simulink model "sampleModel25"  (Simulink 9.1)
settings: Solver=VariableStepAuto  StartTime=0.0  StopTime=10.0  RelTol=1e-3
undefined symbols (not defined in the file): DiscIntNeverNeededParam, Newton, Raphson
libraries: simulink x56
(part 1 of 2)
settings Model: SuppressorTable="22 serialization::archive 11 0 6 0 0 2 8 0 0 0 0 6 0 0 1 0 21 sampleModel25/cfblk71 0 6 0 0 2 8 0 0 0 0 6 41 Simulink:DataType:WarningOverFlowDetected 0 0 0 6 0  0  0 0 0 0 8 20160523 0 0 0 10 57 55 0 1 40 SimulinkFixedPoint:util:Overflowoccurred 0 0 0  0  8 20160523 0 10 57 55 0 1 1 0 21 sampleModel25/cfblk75 2 8 0 41 Simulink:DataType:WarningOverFlowDetected 0 0 0  0  8 20160608 0 15 23 17 0 1 40 SimulinkFixedPoint:util:Overflowoccurred 0 0 0  0  8 20160608 0 15 23 17 0 1"  Creator=DELL  LastModifiedBy=DELL
settings DataIOCC: SaveFormat=Dataset
settings OptimizationCC: LifeSpan=auto
settings DebuggingCC: UnderspecifiedInitializationDetection=Simplified  MergeDetectMultiDrivingBlocksExec=error  SFUnexpectedBacktrackingDiag=error  SFNoUnconditionalDefaultTransitionDiag=error  SFExecutionAtInitializationDiag=warning
settings HardwareCC: ProdBitPerPointer=64  ProdBitPerSizeT=64  ProdBitPerPtrDiffT=64  ProdLargestAtomicFloat=Float  ProdIntDivRoundTo=Zero  ProdEndianess=LittleEndian  ProdWordSize=64  ProdHWDeviceType=Intel->x86-64 (Windows64)
settings ModelReferenceCC: PropagateSignalLabelsOutOfModel=on
settings CodeAppCC: StateflowObjectComments=off
settings GRTTargetCC: TargetLangStandard=C99 (ISO)  CombineOutputUpdateFcns=on  GRTInterface=off
settings ConfigComp: CovMetricSettings=dwe  CovHtmlReporting=off  CovSaveCumulativeToWorkspaceVar=off  CovSaveSingleToWorkspaceVar=off  CovExternalEMLEnable=on

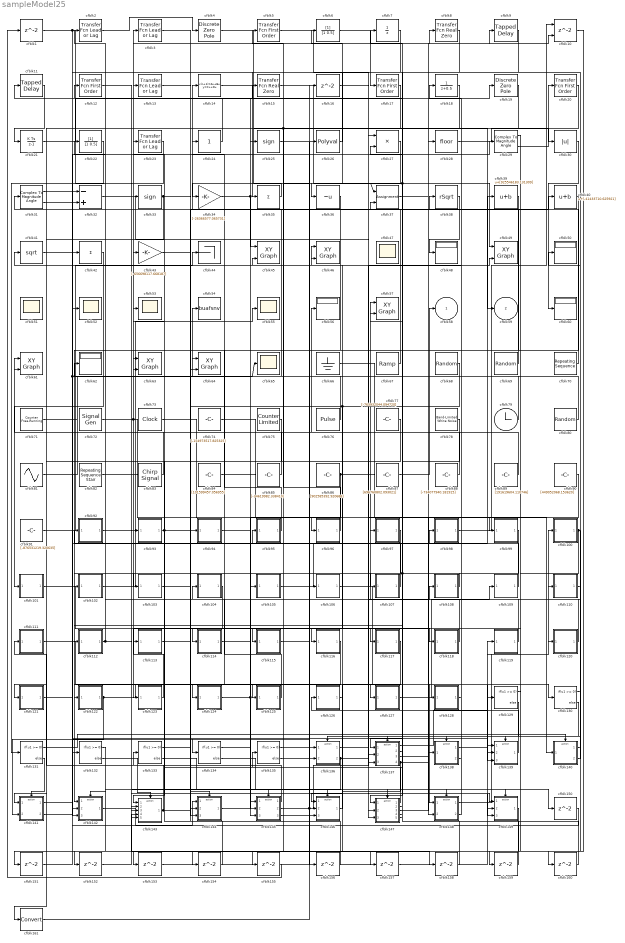
== system sampleModel25 ==
  cfblk{1,16,150..160} (13 alike) : Delay  SampleTime=1
  cfblk10 : Delay  ShowEnablePort=on  SampleTime=1
      settings: InputPortMap=u0,e6
  cfblk100 : Subsystem
  cfblk101 : Subsystem
  cfblk102 : Subsystem
  cfblk103 : Subsystem
  cfblk104 : Subsystem
  cfblk105 : Subsystem
  cfblk106 : Subsystem
  cfblk107 : Subsystem
  cfblk108 : Subsystem
  cfblk109 : Subsystem
  cfblk11 : simulink/Discrete/Tapped Delay  vinit=0.0  samptime=-1  NumDelays=1  DelayOrder=Oldest  includeCurrent=off
  cfblk110 : Subsystem
  cfblk111 : Subsystem
  cfblk112 : Subsystem
  cfblk113 : Subsystem
  cfblk114 : Subsystem
  cfblk115 : Subsystem
  cfblk116 : Subsystem
  cfblk117 : Subsystem
  cfblk118 : Subsystem
  cfblk119 : Subsystem
  cfblk{5,12,17,20} (4 alike) : simulink/Discrete/Transfer Fcn First Order  PoleZ=0.95  ICPrevOutput=0.0  DoSatur=off
      settings: SourceProductName=Simulink
  cfblk120 : Subsystem
  cfblk121 : Subsystem
  cfblk122 : Subsystem
  cfblk123 : Subsystem
  cfblk124 : Subsystem
  cfblk125 : Subsystem
  cfblk126 : Subsystem
  cfblk127 : Subsystem
  cfblk128 : Subsystem
  cfblk{129..135} (7 alike) : If  IfExpression=u1 >= 0  SampleTime=1
  cfblk{2..3,13,23} (4 alike) : simulink/Discrete/Transfer Fcn Lead or Lag  PoleZ=0.95  ZeroZ=0.75  ICPrevOutput=0.0  ICPrevInput=0.0  DoSatur=off
      settings: SourceProductName=Simulink  SourceProductBaseCode=SL
  cfblk136 : Subsystem  TreatAsAtomicUnit=on
  cfblk137 : Subsystem  TreatAsAtomicUnit=on
  cfblk138 : Subsystem  TreatAsAtomicUnit=on
  cfblk139 : Subsystem  TreatAsAtomicUnit=on
  cfblk14 : DiscreteStateSpace
  cfblk140 : Subsystem  TreatAsAtomicUnit=on
  cfblk141 : Subsystem  TreatAsAtomicUnit=on
  cfblk142 : Subsystem  TreatAsAtomicUnit=on
  cfblk143 : Subsystem  TreatAsAtomicUnit=on
  cfblk144 : Subsystem  TreatAsAtomicUnit=on
  cfblk145 : Subsystem  TreatAsAtomicUnit=on
  cfblk146 : Subsystem  TreatAsAtomicUnit=on
  cfblk147 : Subsystem  TreatAsAtomicUnit=on
  cfblk148 : Subsystem  TreatAsAtomicUnit=on
  cfblk149 : Subsystem  TreatAsAtomicUnit=on
  cfblk15 : simulink/Discrete/Transfer Fcn Real Zero  ZeroZ=0.75  ICPrevInput=0.0  DoSatur=off
      settings: SourceProductName=Simulink  SourceProductBaseCode=SL
  cfblk161 : DataTypeConversion
  cfblk18 : DiscreteTransferFcn  SampleTime=1
  cfblk19 : DiscreteZeroPole  Poles=[0 0.5]  Gain=1
  cfblk21 : DiscreteIntegrator  ICPrevOutput=DiscIntNeverNeededParam  ICPrevScaledInput=DiscIntNeverNeededParam
  cfblk22 : DiscreteFilter  SampleTime=1
  cfblk24 : simulink/Math Operations/Slider Gain  gain=1  low=0  high=2
  cfblk25 : Signum
  cfblk26 : Polyval  Coefs=[ +2.081618890e-019, -1.441693666e-014, +4.719686976e-010, -8.536869453e-006, +1.621573104e-001, -8.087801117e+001 ]
  cfblk27 : Product  Inputs=**
  cfblk28 : Rounding
  cfblk29 : ComplexToMagnitudeAngle
  cfblk30 : Abs
  cfblk31 : ComplexToMagnitudeAngle
  cfblk32 : Sum  Inputs=-+
  cfblk33 : Signum
  cfblk34 : Gain  Gain=[-26366577.065731]
  cfblk35 : Sum  Inputs=+
  cfblk36 : UnaryMinus
  cfblk37 : Assignment  DiagnosticForDimensions=Warning  IndexOptions=Index vector (dialog)  Indices=1  OutputSizes=1
  cfblk38 : Sqrt  Operator=rSqrt  AlgorithmType=Newton-Raphson  SaturateOnIntegerOverflow=on
  cfblk39 : Bias  Bias=[925546183.131309]
  cfblk4 : DiscreteZeroPole  Poles=[0 0.5]  Gain=1
  cfblk40 : Bias  Bias=[-41433710.625921]
  cfblk41 : Sqrt  SaturateOnIntegerOverflow=on
  cfblk42 : Sum  Inputs=+
  cfblk43 : Gain  Gain=[-656698117.668187]
  cfblk44 : Terminator
  cfblk{45..46,49,57,61,63..64} (7 alike) : simulink/Sinks/XY Graph  xmin=-1  xmax=1  ymin=-1  ymax=1  st=-1
  cfblk{47,51..53,55,65} (6 alike) : Scope
      cfblk47 settings: Floating=on
      cfblk51 settings: Floating=on
  cfblk{48,50,56,60,62} (5 alike) : Display
  cfblk54 : ToWorkspace  VariableName=buafsnv  SaveFormat=Timeseries  SampleTime=-1
  cfblk6 : DiscreteFilter  SampleTime=1
  cfblk66 : Ground
  cfblk67 : simulink/Sources/Ramp  slope=[-6660.287540]  start=[42.402659]  InitialOutput=[-402163.299320]
  cfblk68 : RandomNumber  Mean=[16622.165096]  Variance=[97213.791717]  Seed=[859309600.000000]  SampleTime=0.1
  cfblk69 : RandomNumber  Mean=[44255.963049]  Variance=[67191.453898]  Seed=[798976347.000000]  SampleTime=0.1
  cfblk7 : UnitDelay
  cfblk70 : simulink/Sources/Repeating Sequence  rep_seq_t=[0 2]  rep_seq_y=[609037232.242526, -300108006.240648]
  cfblk71 : simulink/Sources/Counter Free-Running  NumBits=[2.000000]  tsamp=-1
  cfblk72 : SignalGenerator  Amplitude=[112405273.482846]  Units=rad/sec
  cfblk73 : DigitalClock
  cfblk74 : Constant  Value=[-154973517.825325]  SampleTime=1
  cfblk75 : simulink/Sources/Counter Limited  uplimit=[847.000000]  tsamp=-1
  cfblk76 : DiscretePulseGenerator  PulseType=Time based  Amplitude=[742875642.850489]  Period=[94831116.879649]  PulseWidth=5  PhaseDelay=[9.000000]
  cfblk77 : Constant  Value=[-765932044.094720]  SampleTime=1
  cfblk78 : simulink/Sources/Band-Limited White Noise  Cov=[6434497848.935465]  Ts=0.1  seed=[689213271.000000]
  cfblk79 : Clock
  cfblk8 : simulink/Discrete/Transfer Fcn Real Zero  ZeroZ=0.75  ICPrevInput=0.0  DoSatur=off
      settings: SourceProductName=Simulink  SourceProductBaseCode=SL
  cfblk80 : UniformRandomNumber  Minimum=[-2239471762.590870]  Maximum=[3133993645.558202]  Seed=[35655038.000000]  SampleTime=0.1
  cfblk81 : Sin  Amplitude=[-757481692.637646]  Bias=[-486053189.410621]  SampleTime=0
  cfblk82 : simulink/Sources/Repeating Sequence Stair  OutValues=[-214144912.512597, 953066153.910106]  tsamp=-1  OutMin=[]  OutMax=[]  OutDataTypeStr=double  OutputDataTypeScalingMode=double  OutDataType=fixdt(0,8)  ConRadixGroup=Best Precision: Vector-wise  OutScaling=2^-12
  cfblk83 : simulink/Sources/Chirp Signal  f1=[-335183316.945811]  T=[114581751.178912]  f2=[539771071.082226]
  cfblk84 : Constant  Value=[101599457.056955]  SampleTime=1
  cfblk85 : Constant  Value=[-34619982.338410]  SampleTime=1
  cfblk86 : Constant  Value=[902585392.920688]  SampleTime=1
  cfblk87 : Constant  Value=[696760802.093021]  SampleTime=1
  cfblk88 : Constant  Value=[-734077940.181915]  SampleTime=1
  cfblk89 : Constant  Value=[191619604.110746]  SampleTime=1
  cfblk9 : simulink/Discrete/Tapped Delay  vinit=0.0  samptime=-1  NumDelays=1  DelayOrder=Oldest  includeCurrent=off
  cfblk90 : Constant  Value=[449052068.153620]  SampleTime=1
  cfblk91 : Constant  Value=[-876531219.320635]  SampleTime=1
  cfblk92 : Subsystem
  cfblk93 : Subsystem
  cfblk94 : Subsystem
  cfblk95 : Subsystem
  cfblk96 : Subsystem
  cfblk97 : Subsystem
  cfblk98 : Subsystem
  cfblk99 : Subsystem
  cfblk58 : Outport
  cfblk59 : Outport  Port=2
  wires:
  cfblk107/1(cfblk2) -> cfblk95/1(cfblk1)
  cfblk29/1 -> cfblk114/1(cfblk1)
  cfblk88/1 -> cfblk61/1
  cfblk102/1(cfblk2) -> cfblk55/1
  cfblk99/1(cfblk2) -> cfblk142/1(cfblk1), cfblk143/5(cfblk16)
  cfblk29/2 -> cfblk20/1
  cfblk38/1 -> cfblk48/1
  cfblk148/1(cfblk2) -> cfblk100/1(cfblk1)
  cfblk140/1(cfblk2) -> cfblk35/1
  cfblk79/1 -> cfblk14/1
  cfblk122/1(cfblk2) -> cfblk127/1(cfblk1), cfblk141/2(cfblk10)
  cfblk34/1 -> cfblk45/1, cfblk19/1
  cfblk148/2(cfblk9) -> cfblk45/2
  cfblk120/1(cfblk2) -> cfblk57/1
  cfblk72/1 -> cfblk8/1, cfblk106/1(cfblk1)
  cfblk67/1 -> cfblk3/1
  cfblk89/1 -> cfblk56/1
  cfblk78/1 -> cfblk137/1(cfblk1)
  cfblk104/1(cfblk2) -> cfblk123/1(cfblk1)
  cfblk22/1 -> cfblk131/1
  cfblk14/1 -> cfblk136/1(cfblk1)
  cfblk15/1 -> cfblk49/1
  cfblk8/1 -> cfblk147/1(cfblk1)
  cfblk116/1(cfblk2) -> cfblk122/1(cfblk1)
  cfblk70/1 -> cfblk38/1
  cfblk74/1 -> cfblk96/1(cfblk1)
  cfblk115/1(cfblk2) -> cfblk16/1
  cfblk127/1(cfblk2) -> cfblk109/1(cfblk1)
  cfblk77/1 -> cfblk143/1(cfblk1)
  cfblk9/1 -> cfblk36/1
  cfblk123/1(cfblk2) -> cfblk43/1
  cfblk145/1(cfblk2) -> cfblk113/1(cfblk1)
  cfblk6/1 -> cfblk17/1
  cfblk125/1(cfblk2) -> cfblk104/1(cfblk1)
  cfblk42/1 -> cfblk101/1(cfblk1)
  cfblk32/1 -> cfblk147/2(cfblk12)
  cfblk90/1 -> cfblk147/3(cfblk13)
  cfblk139/1(cfblk2) -> cfblk57/2
  cfblk141/1(cfblk2) -> cfblk63/1
  cfblk17/1 -> cfblk142/3(cfblk10)
  cfblk101/1(cfblk2) -> cfblk118/1(cfblk1)
  cfblk19/1 -> cfblk121/1(cfblk1)
  cfblk106/1(cfblk2) -> cfblk148/1(cfblk1)
  cfblk5/1 -> cfblk137/2(cfblk12)
  cfblk83/1 -> cfblk61/2
  cfblk141/2(cfblk11) -> cfblk97/1(cfblk1)
  cfblk137/1(cfblk2) -> cfblk119/1(cfblk1)
  cfblk11/1 -> cfblk21/1
  cfblk28/1 -> cfblk30/1
  cfblk105/1(cfblk2) -> cfblk39/1
  cfblk30/1 -> cfblk60/1
  cfblk31/1 -> cfblk134/1
  cfblk103/1(cfblk2) -> cfblk115/1(cfblk1)
  cfblk114/1(cfblk2) -> cfblk25/1
  cfblk111/1(cfblk2) -> cfblk139/1(cfblk1)
  cfblk110/1(cfblk2) -> cfblk50/1
  cfblk142/1(cfblk2) -> cfblk144/1(cfblk1)
  cfblk3/1 -> cfblk94/1(cfblk1)
  cfblk26/1 -> cfblk6/1
  cfblk91/1 -> cfblk44/1
  cfblk140/2(cfblk12) -> cfblk110/1(cfblk1)
  cfblk137/2(cfblk14) -> cfblk126/1(cfblk1)
  cfblk20/1 -> cfblk107/1(cfblk1), cfblk37/1
  cfblk124/1(cfblk2) -> cfblk105/1(cfblk1), cfblk149/1(cfblk1)
  cfblk119/1(cfblk2) -> cfblk53/1
  cfblk2/1 -> cfblk4/1
  cfblk41/1 -> cfblk42/1
  cfblk35/1 -> cfblk34/1
  cfblk82/1 -> cfblk140/1(cfblk1)
  cfblk109/1(cfblk2) -> cfblk7/1
  cfblk145/2(cfblk13) -> cfblk108/1(cfblk1)
  cfblk39/1 -> cfblk112/1(cfblk1)
  cfblk13/1 -> cfblk130/1
  cfblk69/1 -> cfblk31/1
  cfblk95/1(cfblk2) -> cfblk24/1
  cfblk1/1 -> cfblk93/1(cfblk1), cfblk139/3(cfblk16)
  cfblk43/1 -> cfblk117/1(cfblk1)
  cfblk76/1 -> cfblk62/1
  cfblk108/1(cfblk2) -> cfblk103/1(cfblk1)
  cfblk98/1(cfblk2) -> cfblk10/1
  cfblk4/1 -> cfblk59/1
  cfblk85/1 -> cfblk2/1
  cfblk113/1(cfblk2) -> cfblk136/2(cfblk15)
  cfblk40/1 -> cfblk124/1(cfblk1)
  cfblk18/1 -> cfblk143/2(cfblk13), cfblk125/1(cfblk1)
  cfblk97/1(cfblk2) -> cfblk102/1(cfblk1)
  cfblk100/1(cfblk2) -> cfblk159/1, cfblk160/1
  cfblk117/1(cfblk2) -> cfblk146/1(cfblk1)
  cfblk23/1 -> cfblk143/3(cfblk14)
  cfblk86/1 -> cfblk128/1(cfblk1), cfblk145/3(cfblk12)
  cfblk93/1(cfblk2) -> cfblk23/1, cfblk137/3(cfblk13)
  cfblk21/1 -> cfblk15/1
  cfblk147/1(cfblk2) -> cfblk63/2
  cfblk147/2(cfblk14) -> cfblk13/1
  cfblk147/3(cfblk15) -> cfblk138/1(cfblk1)
  cfblk94/1(cfblk2) -> cfblk145/1(cfblk1)
  cfblk66/1 -> cfblk148/2(cfblk8)
  cfblk87/1 -> cfblk58/1
  cfblk71/1 -> cfblk54/1
  cfblk68/1 -> cfblk116/1(cfblk1), cfblk144/3(cfblk17)
  cfblk136/1(cfblk2) -> cfblk49/2
  cfblk118/1(cfblk2) -> cfblk22/1
  cfblk143/1(cfblk2) -> cfblk40/1, cfblk111/1(cfblk1)
  cfblk128/1(cfblk2) -> cfblk18/1
  cfblk80/1 -> cfblk33/1
  cfblk121/1(cfblk2) -> cfblk65/1, cfblk29/1
  cfblk7/1 -> cfblk32/2
  cfblk33/1 -> cfblk141/1(cfblk1), cfblk37/2
  cfblk81/1 -> cfblk64/1
  cfblk84/1 -> cfblk99/1(cfblk1)
  cfblk31/2 -> cfblk52/1
  cfblk16/1 -> cfblk27/1
  cfblk144/1(cfblk2) -> cfblk98/1(cfblk1)
  cfblk96/1(cfblk2) -> cfblk5/1
  cfblk147/4(cfblk16) -> cfblk27/2
  cfblk146/1(cfblk2) -> cfblk46/1
  cfblk24/1 -> cfblk11/1
  cfblk37/1 -> cfblk9/1
  cfblk126/1(cfblk2) -> cfblk46/2
  cfblk147/5(cfblk17) -> cfblk92/1(cfblk1)
  cfblk73/1 -> cfblk146/2(cfblk10), cfblk146/3(cfblk11)
  cfblk136/2(cfblk16) -> cfblk149/3(cfblk13), cfblk152/1
  cfblk138/1(cfblk2) -> cfblk120/1(cfblk1)
  cfblk137/3(cfblk15) -> cfblk28/1
  cfblk36/1 -> cfblk64/2
  cfblk138/2(cfblk7) -> cfblk41/1
  cfblk137/4(cfblk16) -> cfblk10/2, cfblk154/1
  cfblk112/1(cfblk2) -> cfblk12/1, cfblk145/2(cfblk11)
  cfblk129/1 -> cfblk136/Action
  cfblk129/2 -> cfblk137/Action
  cfblk130/1 -> cfblk138/Action
  cfblk130/2 -> cfblk139/Action
  cfblk131/1 -> cfblk140/Action
  cfblk131/2 -> cfblk141/Action
  cfblk132/1 -> cfblk142/Action
  cfblk132/2 -> cfblk143/Action
  cfblk133/1 -> cfblk144/Action
  cfblk133/2 -> cfblk145/Action
  cfblk134/1 -> cfblk146/Action
  cfblk134/2 -> cfblk147/Action
  cfblk135/1 -> cfblk148/Action
  cfblk135/2 -> cfblk149/Action
  cfblk12/1 -> cfblk150/1
  cfblk150/1 -> cfblk142/2(cfblk9)
  cfblk10/1 -> cfblk151/1
  cfblk151/1 -> cfblk132/1
  cfblk152/1 -> cfblk143/4(cfblk15)
  cfblk149/1(cfblk2) -> cfblk153/1
  cfblk153/1 -> cfblk129/1
  cfblk154/1 -> cfblk144/2(cfblk16)
  cfblk27/1 -> cfblk155/1
  cfblk155/1 -> cfblk1/1
  cfblk145/3(cfblk14) -> cfblk156/1
  cfblk156/1 -> cfblk133/1
  cfblk25/1 -> cfblk157/1
  cfblk157/1 -> cfblk139/2(cfblk15)
  cfblk92/1(cfblk2) -> cfblk158/1
  cfblk158/1 -> cfblk32/1
  cfblk159/1 -> cfblk135/1
  cfblk160/1 -> cfblk149/2(cfblk12)
  cfblk75/1 -> cfblk161/1
  cfblk161/1 -> cfblk26/1

== system sampleModel25/cfblk100 ==
  cfblk1 : Inport
  cfblk2 : Outport
  wires:
  cfblk1/1 -> cfblk2/1

== system sampleModel25/cfblk101 ==
  cfblk1 : Inport
  cfblk2 : Outport
  wires:
  cfblk1/1 -> cfblk2/1

== system sampleModel25/cfblk102 ==
  cfblk1 : Inport
  cfblk2 : Outport
  wires:
  cfblk1/1 -> cfblk2/1

== system sampleModel25/cfblk103 ==
  cfblk1 : Inport
  cfblk2 : Outport
  wires:
  cfblk1/1 -> cfblk2/1

== system sampleModel25/cfblk104 ==
  cfblk1 : Inport
  cfblk2 : Outport
  wires:
  cfblk1/1 -> cfblk2/1

== system sampleModel25/cfblk105 ==
  cfblk1 : Inport
  cfblk2 : Outport
  wires:
  cfblk1/1 -> cfblk2/1

== system sampleModel25/cfblk106 ==
  cfblk1 : Inport
  cfblk2 : Outport
  wires:
  cfblk1/1 -> cfblk2/1

== system sampleModel25/cfblk107 ==
  cfblk1 : Inport
  cfblk2 : Outport
  wires:
  cfblk1/1 -> cfblk2/1

== system sampleModel25/cfblk108 ==
  cfblk1 : Inport
  cfblk2 : Outport
  wires:
  cfblk1/1 -> cfblk2/1

== system sampleModel25/cfblk109 ==
  cfblk1 : Inport
  cfblk2 : Outport
  wires:
  cfblk1/1 -> cfblk2/1

== system sampleModel25/cfblk110 ==
  cfblk1 : Inport
  cfblk2 : Outport
  wires:
  cfblk1/1 -> cfblk2/1

== system sampleModel25/cfblk111 ==
  cfblk1 : Inport
  cfblk2 : Outport
  wires:
  cfblk1/1 -> cfblk2/1

== system sampleModel25/cfblk112 ==
  cfblk1 : Inport
  cfblk2 : Outport
  wires:
  cfblk1/1 -> cfblk2/1

== system sampleModel25/cfblk113 ==
  cfblk1 : Inport
  cfblk2 : Outport
  wires:
  cfblk1/1 -> cfblk2/1

== system sampleModel25/cfblk114 ==
  cfblk1 : Inport
  cfblk2 : Outport
  wires:
  cfblk1/1 -> cfblk2/1

== system sampleModel25/cfblk115 ==
  cfblk1 : Inport
  cfblk2 : Outport
  wires:
  cfblk1/1 -> cfblk2/1

== system sampleModel25/cfblk116 ==
  cfblk1 : Inport
  cfblk2 : Outport
  wires:
  cfblk1/1 -> cfblk2/1

== system sampleModel25/cfblk117 ==
  cfblk1 : Inport
  cfblk2 : Outport
  wires:
  cfblk1/1 -> cfblk2/1

== system sampleModel25/cfblk118 ==
  cfblk1 : Inport
  cfblk2 : Outport
  wires:
  cfblk1/1 -> cfblk2/1

== system sampleModel25/cfblk119 ==
  cfblk1 : Inport
  cfblk2 : Outport
  wires:
  cfblk1/1 -> cfblk2/1

== system sampleModel25/cfblk120 ==
  cfblk1 : Inport
  cfblk2 : Outport
  wires:
  cfblk1/1 -> cfblk2/1

== system sampleModel25/cfblk121 ==
  cfblk1 : Inport
  cfblk2 : Outport
  wires:
  cfblk1/1 -> cfblk2/1

== system sampleModel25/cfblk122 ==
  cfblk1 : Inport
  cfblk2 : Outport
  wires:
  cfblk1/1 -> cfblk2/1

== system sampleModel25/cfblk123 ==
  cfblk1 : Inport
  cfblk2 : Outport
  wires:
  cfblk1/1 -> cfblk2/1

== system sampleModel25/cfblk124 ==
  cfblk1 : Inport
  cfblk2 : Outport
  wires:
  cfblk1/1 -> cfblk2/1

== system sampleModel25/cfblk125 ==
  cfblk1 : Inport
  cfblk2 : Outport
  wires:
  cfblk1/1 -> cfblk2/1

== system sampleModel25/cfblk126 ==
  cfblk1 : Inport
  cfblk2 : Outport
  wires:
  cfblk1/1 -> cfblk2/1

== system sampleModel25/cfblk127 ==
  cfblk1 : Inport
  cfblk2 : Outport
  wires:
  cfblk1/1 -> cfblk2/1

== system sampleModel25/cfblk128 ==
  cfblk1 : Inport
  cfblk2 : Outport
  wires:
  cfblk1/1 -> cfblk2/1

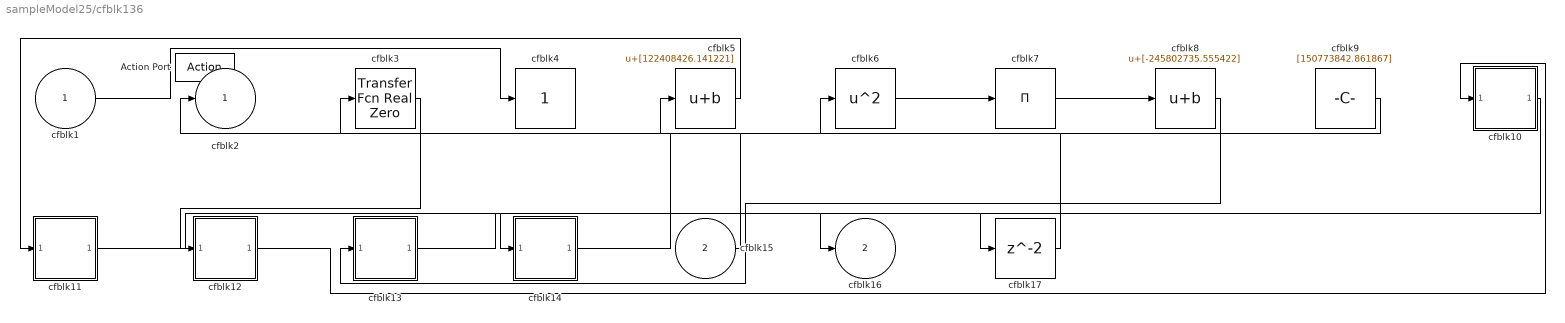
== system sampleModel25/cfblk136 ==
  cfblk1 : Inport
  cfblk15 : Inport  Port=2
  Action Port : ActionPort  ActionType=then
  cfblk10 : Subsystem
  cfblk11 : Subsystem
  cfblk12 : Subsystem
  cfblk13 : Subsystem
  cfblk14 : Subsystem
  cfblk17 : Delay
  cfblk3 : simulink/Discrete/Transfer Fcn Real Zero  ZeroZ=0.75  ICPrevInput=0.0  DoSatur=off
      settings: SourceProductName=Simulink  SourceProductBaseCode=SL
  cfblk4 : simulink/Math Operations/Slider Gain  gain=1  low=0  high=2
  cfblk5 : Bias  Bias=[122408426.141221]
  cfblk6 : Math  Operator=square  SaturateOnIntegerOverflow=on
  cfblk7 : Product  Inputs=*
  cfblk8 : Bias  Bias=[-245802735.555422]
  cfblk9 : Constant  Value=[150773842.861867]  SampleTime=1
  cfblk2 : Outport
  cfblk16 : Outport  Port=2
  wires:
  cfblk10/1(cfblk2) -> cfblk16/1
  cfblk14/1(cfblk2) -> cfblk6/1
  cfblk11/1(cfblk2) -> cfblk14/1(cfblk1)
  cfblk8/1 -> cfblk13/1(cfblk1)
  cfblk3/1 -> cfblk12/1(cfblk1)
  cfblk6/1 -> cfblk7/1
  cfblk1/1 -> cfblk4/1
  cfblk12/1(cfblk2) -> cfblk10/1(cfblk1)
  cfblk7/1 -> cfblk8/1
  cfblk9/1 -> cfblk2/1
  cfblk15/1 -> cfblk3/1
  cfblk5/1 -> cfblk11/1(cfblk1)
  cfblk13/1(cfblk2) -> cfblk17/1
  cfblk17/1 -> cfblk5/1

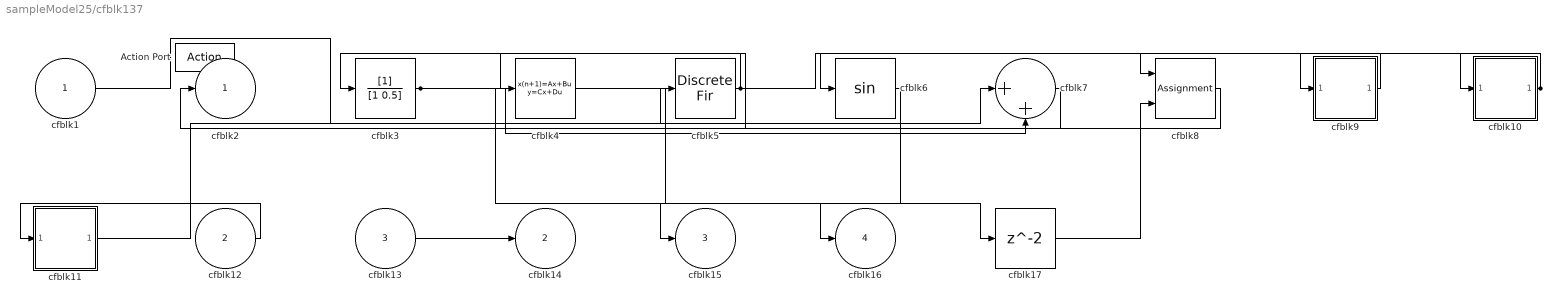
== system sampleModel25/cfblk137 ==
  cfblk1 : Inport
  cfblk12 : Inport  Port=2
  cfblk13 : Inport  Port=3
  Action Port : ActionPort  ActionType=else
  cfblk10 : Subsystem
  cfblk11 : Subsystem
  cfblk17 : Delay
  cfblk3 : DiscreteFilter
  cfblk4 : DiscreteStateSpace  SampleTime=-1
  cfblk5 : DiscreteFir
  cfblk6 : Trigonometry
  cfblk7 : Sum  Inputs=|++
  cfblk8 : Assignment  DiagnosticForDimensions=Warning  IndexOptions=Index vector (dialog)  Indices=1  OutputSizes=1
  cfblk9 : Subsystem
  cfblk2 : Outport
  cfblk14 : Outport  Port=2
  cfblk15 : Outport  Port=3
  cfblk16 : Outport  Port=4
  wires:
  cfblk4/1 -> cfblk16/1
  cfblk9/1(cfblk2) -> cfblk6/1
  cfblk12/1 -> cfblk11/1(cfblk1)
  cfblk8/1 -> cfblk3/1
  cfblk7/1 -> cfblk2/1
  cfblk6/1 -> cfblk15/1
  cfblk1/1 -> cfblk5/1
  cfblk13/1 -> cfblk14/1
  cfblk11/1(cfblk2) -> cfblk7/1
  cfblk10/1(cfblk2) -> cfblk8/1, cfblk9/1(cfblk1)
  cfblk5/1 -> cfblk10/1(cfblk1), cfblk4/1
  cfblk3/1 -> cfblk7/2, cfblk17/1
  cfblk17/1 -> cfblk8/2

== system sampleModel25/cfblk138 ==
  cfblk1 : Inport
  Action Port : ActionPort  ActionType=then
  cfblk3 : Delay
  cfblk4 : Subsystem
  cfblk5 : Subsystem
  cfblk6 : Subsystem
  cfblk2 : Outport
  cfblk7 : Outport  Port=2
  wires:
  cfblk5/1(cfblk2) -> cfblk6/1(cfblk1)
  cfblk4/1(cfblk2) -> cfblk5/1(cfblk1)
  cfblk3/1 -> cfblk4/1(cfblk1)
  cfblk1/1 -> cfblk3/1, cfblk7/1
  cfblk6/1(cfblk2) -> cfblk2/1

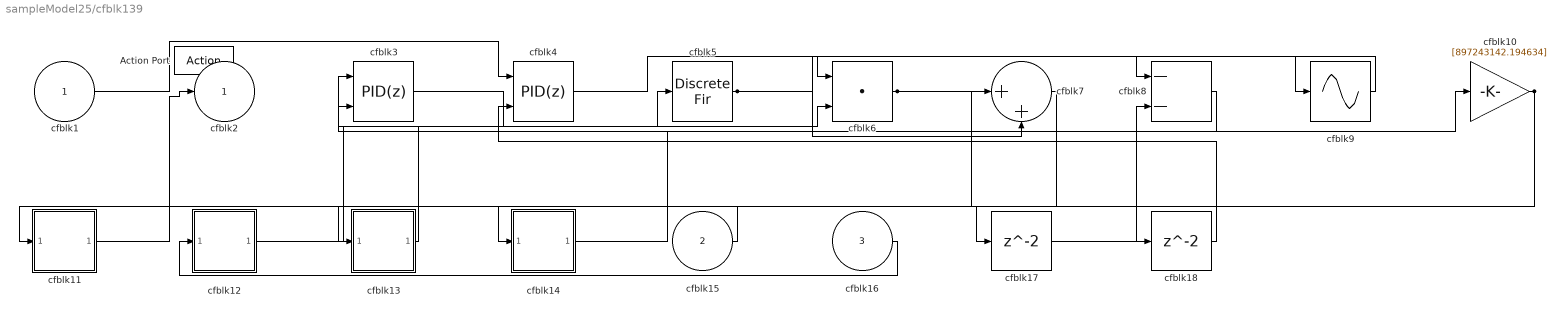
== system sampleModel25/cfblk139 ==
  cfblk1 : Inport
  cfblk15 : Inport  Port=2
  cfblk16 : Inport  Port=3
  Action Port : ActionPort  ActionType=else
  cfblk10 : Gain  Gain=[897243142.194634]
  cfblk11 : Subsystem
  cfblk12 : Subsystem
  cfblk13 : Subsystem
  cfblk14 : Subsystem
  cfblk17 : Delay
  cfblk18 : Delay
  cfblk3 : simulink/Continuous/PID Controller (2DOF)  Controller=PID  TimeDomain=Discrete-time  SampleTime=-1  IntegratorMethod=Forward Euler  FilterMethod=Forward Euler  Form=Parallel  UseFilter=on  ControllerParametersSource=internal  P=1  I=1  D=0  N=100  b=1  c=1  InitialConditionSource=internal  InitialConditionForIntegrator=0  InitialConditionForFilter=0  ExternalReset=none  LimitOutput=off  UpperSaturationLimit=inf  LowerSaturationLimit=-inf  LinearizeAsGain=off  AntiWindupMode=none  Kb=1  TrackingMode=off  Kt=1  PParamMin=[]  PParamMax=[]  IParamMin=[]  IParamMax=[]  DParamMin=[]  DParamMax=[]  NParamMin=[]  NParamMax=[]  bParamMin=[]  bParamMax=[]  cParamMin=[]  cParamMax=[]  KbParamMin=[]  KbParamMax=[]  KtParamMin=[]  KtParamMax=[]  POutMin=[]  POutMax=[]  IOutMin=[]  IOutMax=[]  DOutMin=[]  DOutMax=[]  NOutMin=[]  NOutMax=[]  bOutMin=[]  bOutMax=[]  cOutMin=[]  cOutMax=[]  KbOutMin=[]  KbOutMax=[]  KtOutMin=[]  KtOutMax=[]  IntegratorOutMin=[]  IntegratorOutMax=[]  FilterOutMin=[]  FilterOutMax=[]  SumOutMin=[]  SumOutMax=[]  Sum1OutMin=[]  Sum1OutMax=[]  Sum2OutMin=[]  Sum2OutMax=[]  Sum3OutMin=[]  Sum3OutMax=[]  SumI1OutMin=[]  SumI1OutMax=[]  SumI2OutMin=[]  SumI2OutMax=[]  SumI3OutMin=[]  SumI3OutMax=[]  SumDOutMin=[]  SumDOutMax=[]  SaturationOutMin=[]  SaturationOutMax=[]  IntegratorContinuousStateAttributes=''  IntegratorStateMustResolveToSignalObject=off  IntegratorRTWStateStorageClass=Auto  FilterContinuousStateAttributes=''  FilterStateMustResolveToSignalObject=off  FilterRTWStateStorageClass=Auto  DifferentiatorICPrevScaledInput=0  DifferentiatorOutMin=[]  DifferentiatorOutMax=[]  FilterDiffOutCoefMin=[]  FilterDiffOutCoefMax=[]  SumDenOutMin=[]  SumDenOutMax=[]  SumNumOutMin=[]  SumNumOutMax=[]  ReciprocalOutMin=[]  ReciprocalOutMax=[]  DivideOutMin=[]  DivideOutMax=[]  TunerSelectOption=Transfer Function Based (PID Tuner App)
  cfblk4 : simulink/Continuous/PID Controller (2DOF)  Controller=PID  TimeDomain=Discrete-time  SampleTime=-1  IntegratorMethod=Forward Euler  FilterMethod=Forward Euler  Form=Parallel  UseFilter=on  ControllerParametersSource=internal  P=1  I=1  D=0  N=100  b=1  c=1  InitialConditionSource=internal  InitialConditionForIntegrator=0  InitialConditionForFilter=0  ExternalReset=none  LimitOutput=off  UpperSaturationLimit=inf  LowerSaturationLimit=-inf  LinearizeAsGain=off  AntiWindupMode=none  Kb=1  TrackingMode=off  Kt=1  PParamMin=[]  PParamMax=[]  IParamMin=[]  IParamMax=[]  DParamMin=[]  DParamMax=[]  NParamMin=[]  NParamMax=[]  bParamMin=[]  bParamMax=[]  cParamMin=[]  cParamMax=[]  KbParamMin=[]  KbParamMax=[]  KtParamMin=[]  KtParamMax=[]  POutMin=[]  POutMax=[]  IOutMin=[]  IOutMax=[]  DOutMin=[]  DOutMax=[]  NOutMin=[]  NOutMax=[]  bOutMin=[]  bOutMax=[]  cOutMin=[]  cOutMax=[]  KbOutMin=[]  KbOutMax=[]  KtOutMin=[]  KtOutMax=[]  IntegratorOutMin=[]  IntegratorOutMax=[]  FilterOutMin=[]  FilterOutMax=[]  SumOutMin=[]  SumOutMax=[]  Sum1OutMin=[]  Sum1OutMax=[]  Sum2OutMin=[]  Sum2OutMax=[]  Sum3OutMin=[]  Sum3OutMax=[]  SumI1OutMin=[]  SumI1OutMax=[]  SumI2OutMin=[]  SumI2OutMax=[]  SumI3OutMin=[]  SumI3OutMax=[]  SumDOutMin=[]  SumDOutMax=[]  SaturationOutMin=[]  SaturationOutMax=[]  IntegratorContinuousStateAttributes=''  IntegratorStateMustResolveToSignalObject=off  IntegratorRTWStateStorageClass=Auto  FilterContinuousStateAttributes=''  FilterStateMustResolveToSignalObject=off  FilterRTWStateStorageClass=Auto  DifferentiatorICPrevScaledInput=0  DifferentiatorOutMin=[]  DifferentiatorOutMax=[]  FilterDiffOutCoefMin=[]  FilterDiffOutCoefMax=[]  SumDenOutMin=[]  SumDenOutMax=[]  SumNumOutMin=[]  SumNumOutMax=[]  ReciprocalOutMin=[]  ReciprocalOutMax=[]  DivideOutMin=[]  DivideOutMax=[]  TunerSelectOption=Transfer Function Based (PID Tuner App)
  cfblk5 : DiscreteFir
  cfblk6 : DotProduct  InputSameDT=on  OutDataTypeStr=Inherit: Inherit via internal rule
  cfblk7 : Sum  Inputs=|++
  cfblk8 : Sum  Inputs=--
  cfblk9 : Sin  TimeSource=Use external signal  SampleTime=0
  cfblk2 : Outport
  wires:
  cfblk14/1(cfblk2) -> cfblk10/1
  cfblk12/1(cfblk2) -> cfblk5/1
  cfblk4/1 -> cfblk8/1
  cfblk16/1 -> cfblk12/1(cfblk1)
  cfblk1/1 -> cfblk4/1
  cfblk13/1(cfblk2) -> cfblk3/1
  cfblk9/1 -> cfblk6/1
  cfblk8/1 -> cfblk3/2
  cfblk15/1 -> cfblk14/1(cfblk1)
  cfblk6/1 -> cfblk7/1, cfblk18/1
  cfblk3/1 -> cfblk6/2
  cfblk10/1 -> cfblk13/1(cfblk1), cfblk11/1(cfblk1)
  cfblk5/1 -> cfblk7/2, cfblk9/1
  cfblk11/1(cfblk2) -> cfblk2/1
  cfblk7/1 -> cfblk17/1
  cfblk17/1 -> cfblk8/2
  cfblk18/1 -> cfblk4/2

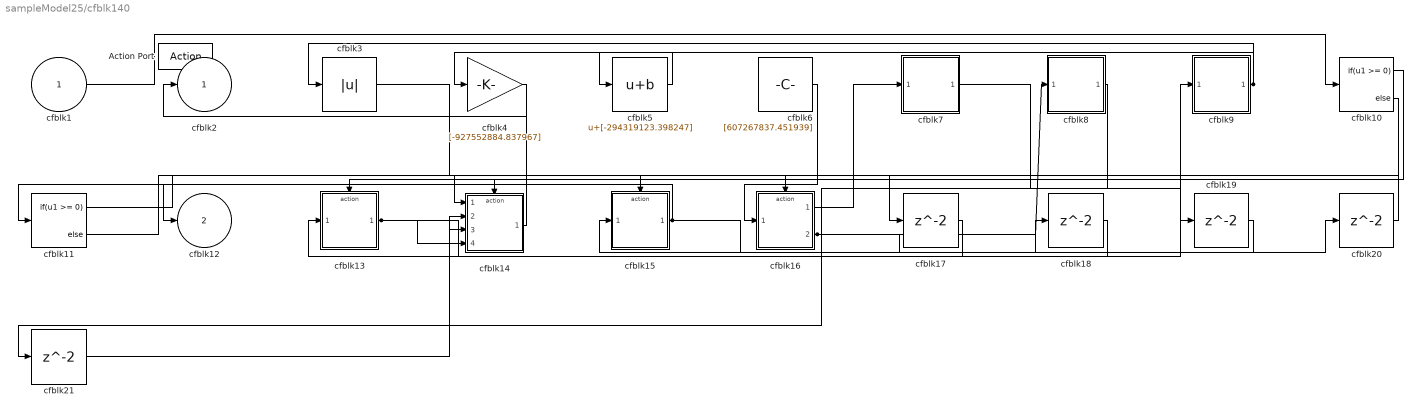
== system sampleModel25/cfblk140 ==
  cfblk1 : Inport
  Action Port : ActionPort  ActionType=then
  cfblk10 : If  IfExpression=u1 >= 0  SampleTime=1
  cfblk11 : If  IfExpression=u1 >= 0  SampleTime=1
  cfblk13 : Subsystem  TreatAsAtomicUnit=on
  cfblk14 : Subsystem  TreatAsAtomicUnit=on
  cfblk15 : Subsystem  TreatAsAtomicUnit=on
  cfblk16 : Subsystem  TreatAsAtomicUnit=on
  cfblk{17..21} (5 alike) : Delay
  cfblk3 : Abs
  cfblk4 : Gain  Gain=[-927552884.837967]
  cfblk5 : Bias  Bias=[-294319123.398247]
  cfblk6 : Constant  Value=[607267837.451939]  SampleTime=1
  cfblk7 : Subsystem
  cfblk8 : Subsystem
  cfblk9 : Subsystem
  cfblk2 : Outport
  cfblk12 : Outport  Port=2
  wires:
  cfblk16/1(cfblk2) -> cfblk7/1(cfblk1)
  cfblk9/1(cfblk2) -> cfblk3/1, cfblk5/1
  cfblk13/1(cfblk2) -> cfblk9/1(cfblk1), cfblk14/4(cfblk12)
  cfblk14/1(cfblk2) -> cfblk2/1
  cfblk15/1(cfblk2) -> cfblk12/1, cfblk18/1
  cfblk6/1 -> cfblk16/1(cfblk1)
  cfblk16/2(cfblk8) -> cfblk8/1(cfblk1), cfblk20/1
  cfblk4/1 -> cfblk11/1
  cfblk1/1 -> cfblk10/1
  cfblk5/1 -> cfblk4/1
  cfblk10/1 -> cfblk13/Action
  cfblk10/2 -> cfblk14/Action
  cfblk11/1 -> cfblk15/Action
  cfblk11/2 -> cfblk16/Action
  cfblk3/1 -> cfblk17/1
  cfblk17/1 -> cfblk14/2(cfblk10)
  cfblk18/1 -> cfblk13/1(cfblk1)
  cfblk7/1(cfblk2) -> cfblk19/1
  cfblk19/1 -> cfblk15/1(cfblk1)
  cfblk20/1 -> cfblk14/1(cfblk1)
  cfblk8/1(cfblk2) -> cfblk21/1
  cfblk21/1 -> cfblk14/3(cfblk11)

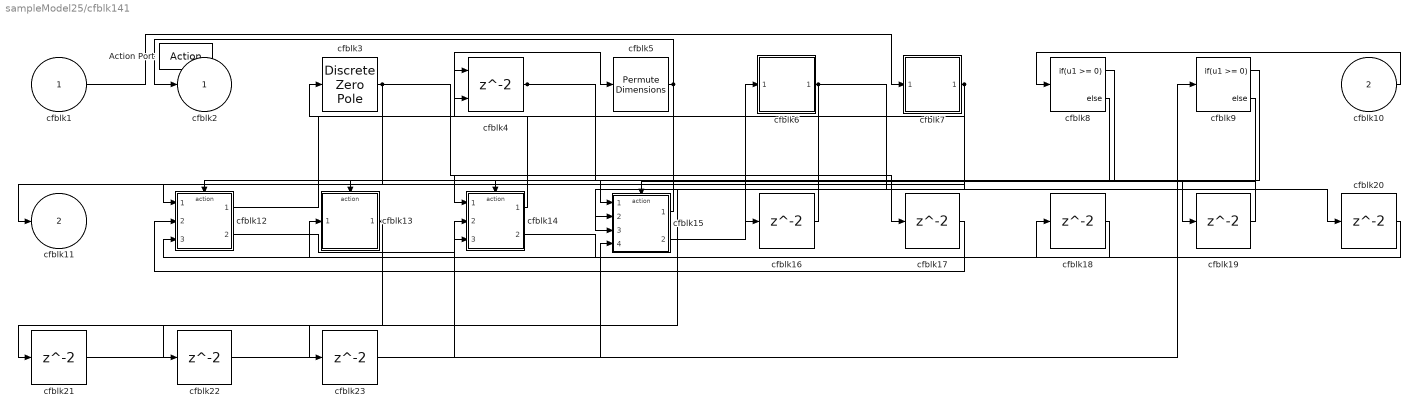
== system sampleModel25/cfblk141 ==
  cfblk1 : Inport
  cfblk10 : Inport  Port=2
  Action Port : ActionPort  ActionType=else
  cfblk12 : Subsystem  TreatAsAtomicUnit=on
  cfblk13 : Subsystem  TreatAsAtomicUnit=on
  cfblk14 : Subsystem  TreatAsAtomicUnit=on
  cfblk15 : Subsystem  TreatAsAtomicUnit=on
  cfblk{16..23} (8 alike) : Delay
  cfblk3 : DiscreteZeroPole  Poles=[0 0.5]  Gain=1  SampleTime=-1
  cfblk4 : Delay  ShowEnablePort=on
      settings: InputPortMap=u0,e6
  cfblk5 : PermuteDimensions
  cfblk6 : Subsystem
  cfblk7 : Subsystem
  cfblk8 : If  IfExpression=u1 >= 0  SampleTime=1
  cfblk9 : If  IfExpression=u1 >= 0  SampleTime=1
  cfblk2 : Outport
  cfblk11 : Outport  Port=2
  wires:
  cfblk13/1(cfblk2) -> cfblk21/1, cfblk22/1
  cfblk5/1 -> cfblk2/1, cfblk15/3(cfblk13)
  cfblk1/1 -> cfblk7/1(cfblk1)
  cfblk10/1 -> cfblk8/1
  cfblk12/1(cfblk2) -> cfblk5/1
  cfblk6/1(cfblk2) -> cfblk20/1, cfblk23/1
  cfblk14/1(cfblk2) -> cfblk3/1
  cfblk4/1 -> cfblk16/1, cfblk19/1
  cfblk12/2(cfblk15) -> cfblk14/2(cfblk15)
  cfblk7/1(cfblk2) -> cfblk12/1(cfblk1), cfblk4/2, cfblk15/2(cfblk12)
  cfblk3/1 -> cfblk11/1, cfblk17/1
  cfblk15/1(cfblk2) -> cfblk4/1
  cfblk15/2(cfblk15) -> cfblk6/1(cfblk1)
  cfblk8/1 -> cfblk12/Action
  cfblk8/2 -> cfblk13/Action
  cfblk9/1 -> cfblk14/Action
  cfblk9/2 -> cfblk15/Action
  cfblk16/1 -> cfblk14/1(cfblk1)
  cfblk17/1 -> cfblk12/2(cfblk13)
  cfblk14/2(cfblk17) -> cfblk18/1
  cfblk18/1 -> cfblk12/3(cfblk14)
  cfblk19/1 -> cfblk15/1(cfblk1)
  cfblk20/1 -> cfblk13/1(cfblk1)
  cfblk21/1 -> cfblk9/1
  cfblk22/1 -> cfblk15/4(cfblk14)
  cfblk23/1 -> cfblk14/3(cfblk16)

== system sampleModel25/cfblk142 ==
  cfblk1 : Inport
  cfblk9 : Inport  Port=2
  cfblk10 : Inport  Port=3
  Action Port : ActionPort  ActionType=then
  cfblk3 : DiscreteZeroPole  Poles=[0 0.5]  Gain=1  SampleTime=-1
  cfblk4 : Squeeze
  cfblk5 : Sqrt  SaturateOnIntegerOverflow=on
  cfblk6 : Sin  TimeSource=Use external signal  SampleTime=0
  cfblk7 : simulink/Math Operations/Slider Gain  gain=1  low=0  high=2
  cfblk8 : Subsystem
  cfblk2 : Outport
  wires:
  cfblk1/1 -> cfblk7/1
  cfblk6/1 -> cfblk5/1
  cfblk9/1 -> cfblk6/1
  cfblk5/1 -> cfblk8/1(cfblk1)
  cfblk8/1(cfblk2) -> cfblk3/1
  cfblk10/1 -> cfblk4/1
  cfblk3/1 -> cfblk2/1

== system sampleModel25/cfblk143 ==
  cfblk1 : Inport
  cfblk13 : Inport  Port=2
  cfblk14 : Inport  Port=3
  cfblk15 : Inport  Port=4
  cfblk16 : Inport  Port=5
  Action Port : ActionPort  ActionType=else
  cfblk10 : Subsystem
  cfblk11 : Subsystem
  cfblk12 : Subsystem
  cfblk17 : Delay
  cfblk3 : UnitDelay  SampleTime=-1
  cfblk4 : simulink/Discrete/Transfer Fcn Lead or Lag  PoleZ=0.95  ZeroZ=0.75  ICPrevOutput=0.0  ICPrevInput=0.0  DoSatur=off
      settings: SourceProductName=Simulink  SourceProductBaseCode=SL
  cfblk5 : simulink/Discrete/Transfer Fcn First Order  PoleZ=0.95  ICPrevOutput=0.0  DoSatur=off
      settings: SourceProductName=Simulink
  cfblk6 : simulink/Discrete/Difference  ICPrevInput=0.0  OutMin=[]  OutMax=[]  OutDataTypeStr=Inherit: Inherit via back propagation  OutDataType=fixdt(1, 16)  OutScaling=2^-10  DoSatur=off
  cfblk7 : DiscreteTransferFcn
  cfblk8 : Squeeze
  cfblk9 : Subsystem
  cfblk2 : Outport
  wires:
  cfblk7/1 -> cfblk9/1(cfblk1)
  cfblk6/1 -> cfblk10/1(cfblk1)
  cfblk15/1 -> cfblk3/1
  cfblk10/1(cfblk2) -> cfblk2/1
  cfblk13/1 -> cfblk5/1
  cfblk9/1(cfblk2) -> cfblk8/1
  cfblk4/1 -> cfblk11/1(cfblk1)
  cfblk1/1 -> cfblk6/1
  cfblk3/1 -> cfblk12/1(cfblk1)
  cfblk5/1 -> cfblk7/1
  cfblk11/1(cfblk2) -> cfblk17/1
  cfblk17/1 -> cfblk4/1

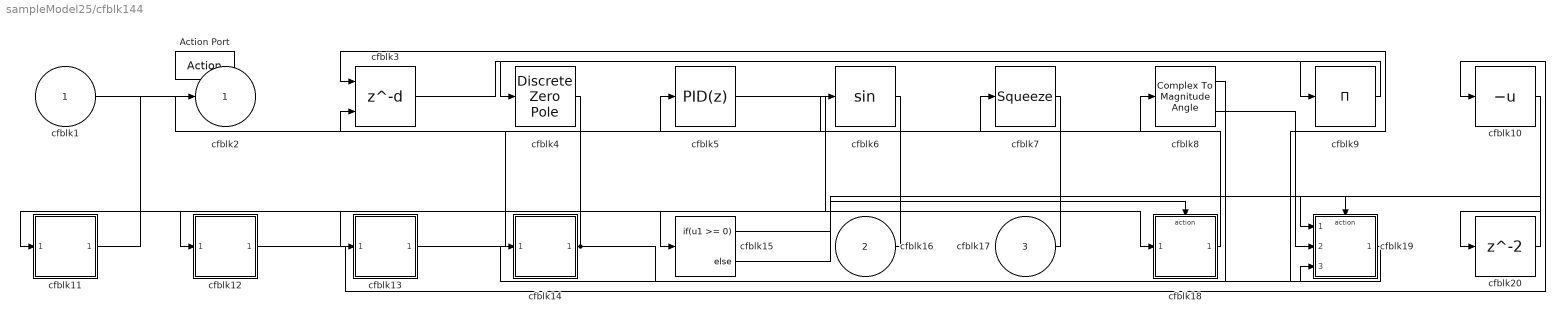
== system sampleModel25/cfblk144 ==
  cfblk1 : Inport
  cfblk16 : Inport  Port=2
  cfblk17 : Inport  Port=3
  Action Port : ActionPort  ActionType=then
  cfblk10 : UnaryMinus
  cfblk11 : Subsystem
  cfblk12 : Subsystem
  cfblk13 : Subsystem
  cfblk14 : Subsystem
  cfblk15 : If  IfExpression=u1 >= 0  SampleTime=1
  cfblk18 : Subsystem  TreatAsAtomicUnit=on
  cfblk19 : Subsystem  TreatAsAtomicUnit=on
  cfblk20 : Delay
  cfblk3 : Delay  DelayLengthSource=Input port
      settings: InputPortMap=u0,p1
  cfblk4 : DiscreteZeroPole  Poles=[0 0.5]  Gain=1  SampleTime=-1
  cfblk5 : simulink/Continuous/PID Controller  Controller=PID  TimeDomain=Discrete-time  SampleTime=-1  IntegratorMethod=Forward Euler  FilterMethod=Forward Euler  Form=Parallel  UseFilter=on  ControllerParametersSource=internal  P=1  I=1  D=0  N=100  InitialConditionSource=internal  InitialConditionForIntegrator=0  InitialConditionForFilter=0  ExternalReset=none  LimitOutput=off  UpperSaturationLimit=inf  LowerSaturationLimit=-inf  LinearizeAsGain=off  AntiWindupMode=none  Kb=1  TrackingMode=off  Kt=1  PParamMin=[]  PParamMax=[]  IParamMin=[]  IParamMax=[]  DParamMin=[]  DParamMax=[]  NParamMin=[]  NParamMax=[]  KbParamMin=[]  KbParamMax=[]  KtParamMin=[]  KtParamMax=[]  POutMin=[]  POutMax=[]  IOutMin=[]  IOutMax=[]  DOutMin=[]  DOutMax=[]  NOutMin=[]  NOutMax=[]  KbOutMin=[]  KbOutMax=[]  KtOutMin=[]  KtOutMax=[]  IntegratorOutMin=[]  IntegratorOutMax=[]  FilterOutMin=[]  FilterOutMax=[]  SumOutMin=[]  SumOutMax=[]  SumI1OutMin=[]  SumI1OutMax=[]  SumI2OutMin=[]  SumI2OutMax=[]  SumI3OutMin=[]  SumI3OutMax=[]  SumDOutMin=[]  SumDOutMax=[]  SaturationOutMin=[]  SaturationOutMax=[]  IntegratorContinuousStateAttributes=''  IntegratorStateMustResolveToSignalObject=off  IntegratorRTWStateStorageClass=Auto  FilterContinuousStateAttributes=''  FilterStateMustResolveToSignalObject=off  FilterRTWStateStorageClass=Auto  DifferentiatorICPrevScaledInput=0  DifferentiatorOutMin=[]  DifferentiatorOutMax=[]  FilterDiffOutCoefMin=[]  FilterDiffOutCoefMax=[]  SumDenOutMin=[]  SumDenOutMax=[]  SumNumOutMin=[]  SumNumOutMax=[]  ReciprocalOutMin=[]  ReciprocalOutMax=[]  DivideOutMin=[]  DivideOutMax=[]  TunerSelectOption=Transfer Function Based (PID Tuner App)
  cfblk6 : Trigonometry
  cfblk7 : Squeeze
  cfblk8 : ComplexToMagnitudeAngle
  cfblk9 : Product  Inputs=*
  cfblk2 : Outport
  wires:
  cfblk11/1(cfblk2) -> cfblk2/1
  cfblk5/1 -> cfblk18/1(cfblk1)
  cfblk4/1 -> cfblk12/1(cfblk1)
  cfblk9/1 -> cfblk4/1
  cfblk13/1(cfblk2) -> cfblk7/1
  cfblk7/1 -> cfblk11/1(cfblk1)
  cfblk1/1 -> cfblk8/1
  cfblk19/1(cfblk2) -> cfblk3/1
  cfblk16/1 -> cfblk5/1
  cfblk8/1 -> cfblk14/1(cfblk1)
  cfblk6/1 -> cfblk15/1
  cfblk17/1 -> cfblk6/1
  cfblk8/2 -> cfblk19/2(cfblk7)
  cfblk14/1(cfblk2) -> cfblk19/3(cfblk8), cfblk13/1(cfblk1)
  cfblk3/1 -> cfblk9/1
  cfblk18/1(cfblk2) -> cfblk3/2
  cfblk12/1(cfblk2) -> cfblk10/1
  cfblk15/1 -> cfblk18/Action
  cfblk15/2 -> cfblk19/Action
  cfblk10/1 -> cfblk20/1
  cfblk20/1 -> cfblk19/1(cfblk1)

== system sampleModel25/cfblk145 ==
  cfblk1 : Inport
  cfblk11 : Inport  Port=2
  cfblk12 : Inport  Port=3
  Action Port : ActionPort  ActionType=else
  cfblk10 : Subsystem
  cfblk15 : Delay
  cfblk3 : DiscreteTransferFcn
  cfblk4 : simulink/Discrete/Difference  ICPrevInput=0.0  OutMin=[]  OutMax=[]  OutDataTypeStr=Inherit: Inherit via back propagation  OutDataType=fixdt(1, 16)  OutScaling=2^-10  DoSatur=off
  cfblk5 : Product  Inputs=*
  cfblk6 : Constant  Value=[-704790414.995481]  SampleTime=1
  cfblk7 : Subsystem
  cfblk8 : Subsystem
  cfblk9 : Subsystem
  cfblk2 : Outport
  cfblk13 : Outport  Port=2
  cfblk14 : Outport  Port=3
  wires:
  cfblk6/1 -> cfblk14/1
  cfblk9/1(cfblk2) -> cfblk7/1(cfblk1)
  cfblk3/1 -> cfblk5/1
  cfblk11/1 -> cfblk9/1(cfblk1)
  cfblk7/1(cfblk2) -> cfblk8/1(cfblk1)
  cfblk8/1(cfblk2) -> cfblk3/1
  cfblk12/1 -> cfblk13/1
  cfblk5/1 -> cfblk2/1
  cfblk4/1 -> cfblk10/1(cfblk1)
  cfblk10/1(cfblk2) -> cfblk15/1
  cfblk15/1 -> cfblk4/1

== system sampleModel25/cfblk146 ==
  cfblk1 : Inport
  cfblk10 : Inport  Port=2
  cfblk11 : Inport  Port=3
  Action Port : ActionPort  ActionType=then
  cfblk3 : simulink/Discrete/Transfer Fcn First Order  PoleZ=0.95  ICPrevOutput=0.0  DoSatur=off
      settings: SourceProductName=Simulink
  cfblk4 : simulink/Math Operations/MinMax Running Resettable  Function=min  vinit=0.0
  cfblk5 : Product
  cfblk6 : Signum
  cfblk7 : simulink/Math Operations/Slider Gain  gain=1  low=0  high=2
  cfblk8 : Constant  Value=[34703357.405781]  SampleTime=1
  cfblk9 : Subsystem
  cfblk2 : Outport
  wires:
  cfblk10/1 -> cfblk6/1
  cfblk8/1 -> cfblk3/1
  cfblk11/1 -> cfblk5/1
  cfblk9/1(cfblk2) -> cfblk5/2
  cfblk4/1 -> cfblk9/1(cfblk1)
  cfblk3/1 -> cfblk4/1
  cfblk7/1 -> cfblk4/2
  cfblk6/1 -> cfblk2/1
  cfblk1/1 -> cfblk7/1

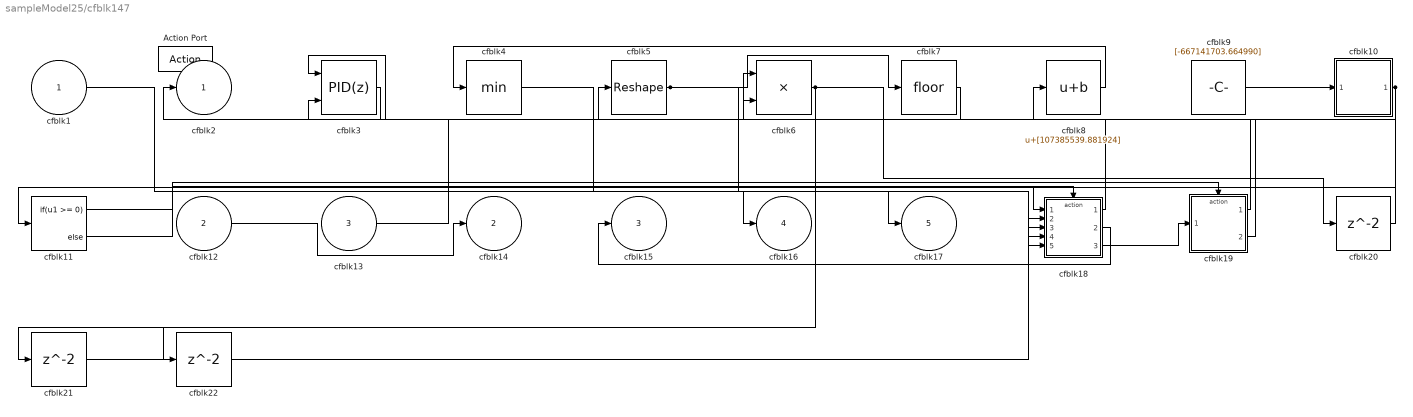
== system sampleModel25/cfblk147 ==
  cfblk1 : Inport
  cfblk12 : Inport  Port=2
  cfblk13 : Inport  Port=3
  Action Port : ActionPort  ActionType=else
  cfblk10 : Subsystem
  cfblk11 : If  IfExpression=u1 >= 0  SampleTime=1
  cfblk18 : Subsystem  TreatAsAtomicUnit=on
  cfblk19 : Subsystem  TreatAsAtomicUnit=on
  cfblk20 : Delay
  cfblk21 : Delay
  cfblk22 : Delay
  cfblk3 : simulink/Continuous/PID Controller (2DOF)  Controller=PID  TimeDomain=Discrete-time  SampleTime=-1  IntegratorMethod=Forward Euler  FilterMethod=Forward Euler  Form=Parallel  UseFilter=on  ControllerParametersSource=internal  P=1  I=1  D=0  N=100  b=1  c=1  InitialConditionSource=internal  InitialConditionForIntegrator=0  InitialConditionForFilter=0  ExternalReset=none  LimitOutput=off  UpperSaturationLimit=inf  LowerSaturationLimit=-inf  LinearizeAsGain=off  AntiWindupMode=none  Kb=1  TrackingMode=off  Kt=1  PParamMin=[]  PParamMax=[]  IParamMin=[]  IParamMax=[]  DParamMin=[]  DParamMax=[]  NParamMin=[]  NParamMax=[]  bParamMin=[]  bParamMax=[]  cParamMin=[]  cParamMax=[]  KbParamMin=[]  KbParamMax=[]  KtParamMin=[]  KtParamMax=[]  POutMin=[]  POutMax=[]  IOutMin=[]  IOutMax=[]  DOutMin=[]  DOutMax=[]  NOutMin=[]  NOutMax=[]  bOutMin=[]  bOutMax=[]  cOutMin=[]  cOutMax=[]  KbOutMin=[]  KbOutMax=[]  KtOutMin=[]  KtOutMax=[]  IntegratorOutMin=[]  IntegratorOutMax=[]  FilterOutMin=[]  FilterOutMax=[]  SumOutMin=[]  SumOutMax=[]  Sum1OutMin=[]  Sum1OutMax=[]  Sum2OutMin=[]  Sum2OutMax=[]  Sum3OutMin=[]  Sum3OutMax=[]  SumI1OutMin=[]  SumI1OutMax=[]  SumI2OutMin=[]  SumI2OutMax=[]  SumI3OutMin=[]  SumI3OutMax=[]  SumDOutMin=[]  SumDOutMax=[]  SaturationOutMin=[]  SaturationOutMax=[]  IntegratorContinuousStateAttributes=''  IntegratorStateMustResolveToSignalObject=off  IntegratorRTWStateStorageClass=Auto  FilterContinuousStateAttributes=''  FilterStateMustResolveToSignalObject=off  FilterRTWStateStorageClass=Auto  DifferentiatorICPrevScaledInput=0  DifferentiatorOutMin=[]  DifferentiatorOutMax=[]  FilterDiffOutCoefMin=[]  FilterDiffOutCoefMax=[]  SumDenOutMin=[]  SumDenOutMax=[]  SumNumOutMin=[]  SumNumOutMax=[]  ReciprocalOutMin=[]  ReciprocalOutMax=[]  DivideOutMin=[]  DivideOutMax=[]  TunerSelectOption=Transfer Function Based (PID Tuner App)
  cfblk4 : MinMax
  cfblk5 : Reshape
  cfblk6 : Product
  cfblk7 : Rounding
  cfblk8 : Bias  Bias=[107385539.881924]
  cfblk9 : Constant  Value=[-667141703.664990]  SampleTime=1
  cfblk2 : Outport
  cfblk14 : Outport  Port=2
  cfblk15 : Outport  Port=3
  cfblk16 : Outport  Port=4
  cfblk17 : Outport  Port=5
  wires:
  cfblk9/1 -> cfblk10/1(cfblk1)
  cfblk3/1 -> cfblk2/1
  cfblk6/1 -> cfblk20/1, cfblk21/1, cfblk22/1
  cfblk1/1 -> cfblk17/1
  cfblk18/1(cfblk2) -> cfblk3/1
  cfblk8/1 -> cfblk4/1
  cfblk5/1 -> cfblk7/1, cfblk18/2(cfblk6), cfblk18/5(cfblk9)
  cfblk19/1(cfblk2) -> cfblk6/1
  cfblk18/2(cfblk10) -> cfblk15/1
  cfblk10/1(cfblk2) -> cfblk18/1(cfblk1), cfblk11/1
  cfblk7/1 -> cfblk3/2
  cfblk19/2(cfblk13) -> cfblk8/1
  cfblk12/1 -> cfblk14/1
  cfblk4/1 -> cfblk16/1
  cfblk13/1 -> cfblk6/2
  cfblk18/3(cfblk11) -> cfblk19/1(cfblk1)
  cfblk11/1 -> cfblk18/Action
  cfblk11/2 -> cfblk19/Action
  cfblk20/1 -> cfblk5/1
  cfblk21/1 -> cfblk18/3(cfblk7)
  cfblk22/1 -> cfblk18/4(cfblk8)

== system sampleModel25/cfblk148 ==
  cfblk1 : Inport
  cfblk8 : Inport  Port=2
  Action Port : ActionPort  ActionType=then
  cfblk10 : Delay
  cfblk3 : Sin  TimeSource=Use external signal  SampleTime=0
  cfblk4 : Reshape
  cfblk5 : Assignment  DiagnosticForDimensions=Warning  IndexOptions=Index vector (dialog)  Indices=1  OutputSizes=1
  cfblk6 : Math  Operator=hypot  SaturateOnIntegerOverflow=on
  cfblk7 : Subsystem
  cfblk2 : Outport
  cfblk9 : Outport  Port=2
  wires:
  cfblk8/1 -> cfblk4/1
  cfblk1/1 -> cfblk5/1
  cfblk6/1 -> cfblk7/1(cfblk1)
  cfblk4/1 -> cfblk6/1
  cfblk3/1 -> cfblk5/2, cfblk6/2
  cfblk5/1 -> cfblk9/1, cfblk2/1
  cfblk7/1(cfblk2) -> cfblk10/1
  cfblk10/1 -> cfblk3/1

== system sampleModel25/cfblk149 ==
  cfblk1 : Inport
  cfblk12 : Inport  Port=2
  cfblk13 : Inport  Port=3
  Action Port : ActionPort  ActionType=else
  cfblk10 : Subsystem
  cfblk11 : Subsystem
  cfblk3 : DiscreteIntegrator  SampleTime=-1  ICPrevOutput=DiscIntNeverNeededParam  ICPrevScaledInput=DiscIntNeverNeededParam
  cfblk4 : Delay  DelayLengthSource=Input port
      settings: InputPortMap=u0,p1
  cfblk5 : Sin  TimeSource=Use external signal  SampleTime=0
  cfblk6 : Product  Inputs=*
  cfblk7 : Constant  Value=[982235476.190691]  SampleTime=1
  cfblk8 : Subsystem
  cfblk9 : Subsystem
  cfblk2 : Outport
  wires:
  cfblk9/1(cfblk2) -> cfblk2/1
  cfblk12/1 -> cfblk4/1
  cfblk5/1 -> cfblk3/1
  cfblk1/1 -> cfblk5/1
  cfblk8/1(cfblk2) -> cfblk6/1
  cfblk3/1 -> cfblk8/1(cfblk1)
  cfblk13/1 -> cfblk4/2
  cfblk10/1(cfblk2) -> cfblk9/1(cfblk1)
  cfblk6/1 -> cfblk11/1(cfblk1)
  cfblk4/1 -> cfblk10/1(cfblk1)

== system sampleModel25/cfblk92 ==
  cfblk1 : Inport
  cfblk2 : Outport
  wires:
  cfblk1/1 -> cfblk2/1

== system sampleModel25/cfblk93 ==
  cfblk1 : Inport
  cfblk2 : Outport
  wires:
  cfblk1/1 -> cfblk2/1

== system sampleModel25/cfblk94 ==
  cfblk1 : Inport
  cfblk2 : Outport
  wires:
  cfblk1/1 -> cfblk2/1

== system sampleModel25/cfblk95 ==
  cfblk1 : Inport
  cfblk2 : Outport
  wires:
  cfblk1/1 -> cfblk2/1

== system sampleModel25/cfblk96 ==
  cfblk1 : Inport
  cfblk2 : Outport
  wires:
  cfblk1/1 -> cfblk2/1

== system sampleModel25/cfblk97 ==
  cfblk1 : Inport
  cfblk2 : Outport
  wires:
  cfblk1/1 -> cfblk2/1

== system sampleModel25/cfblk98 ==
  cfblk1 : Inport
  cfblk2 : Outport
  wires:
  cfblk1/1 -> cfblk2/1

== system sampleModel25/cfblk99 ==
  cfblk1 : Inport
  cfblk2 : Outport
  wires:
  cfblk1/1 -> cfblk2/1

== system sampleModel25/cfblk136/cfblk10 ==
  cfblk1 : Inport
  cfblk2 : Outport
  wires:
  cfblk1/1 -> cfblk2/1

== system sampleModel25/cfblk136/cfblk11 ==
  cfblk1 : Inport
  cfblk2 : Outport
  wires:
  cfblk1/1 -> cfblk2/1

== system sampleModel25/cfblk136/cfblk12 ==
  cfblk1 : Inport
  cfblk2 : Outport
  wires:
  cfblk1/1 -> cfblk2/1

== system sampleModel25/cfblk136/cfblk13 ==
  cfblk1 : Inport
  cfblk2 : Outport
  wires:
  cfblk1/1 -> cfblk2/1

== system sampleModel25/cfblk136/cfblk14 ==
  cfblk1 : Inport
  cfblk2 : Outport
  wires:
  cfblk1/1 -> cfblk2/1

== system sampleModel25/cfblk137/cfblk10 ==
  cfblk1 : Inport
  cfblk2 : Outport
  wires:
  cfblk1/1 -> cfblk2/1

== system sampleModel25/cfblk137/cfblk11 ==
  cfblk1 : Inport
  cfblk2 : Outport
  wires:
  cfblk1/1 -> cfblk2/1

== system sampleModel25/cfblk137/cfblk9 ==
  cfblk1 : Inport
  cfblk2 : Outport
  wires:
  cfblk1/1 -> cfblk2/1

== system sampleModel25/cfblk138/cfblk4 ==
  cfblk1 : Inport
  cfblk2 : Outport
  wires:
  cfblk1/1 -> cfblk2/1

== system sampleModel25/cfblk138/cfblk5 ==
  cfblk1 : Inport
  cfblk2 : Outport
  wires:
  cfblk1/1 -> cfblk2/1

== system sampleModel25/cfblk138/cfblk6 ==
  cfblk1 : Inport
  cfblk2 : Outport
  wires:
  cfblk1/1 -> cfblk2/1

== system sampleModel25/cfblk139/cfblk11 ==
  cfblk1 : Inport
  cfblk2 : Outport
  wires:
  cfblk1/1 -> cfblk2/1

== system sampleModel25/cfblk139/cfblk12 ==
  cfblk1 : Inport
  cfblk2 : Outport
  wires:
  cfblk1/1 -> cfblk2/1

== system sampleModel25/cfblk139/cfblk13 ==
  cfblk1 : Inport
  cfblk2 : Outport
  wires:
  cfblk1/1 -> cfblk2/1

== system sampleModel25/cfblk139/cfblk14 ==
  cfblk1 : Inport
  cfblk2 : Outport
  wires:
  cfblk1/1 -> cfblk2/1

== system sampleModel25/cfblk140/cfblk13 ==
  cfblk1 : Inport
  Action Port : ActionPort  ActionType=then
  cfblk10 : Subsystem
  cfblk11 : Subsystem
  cfblk12 : Subsystem
  cfblk13 : Subsystem
  cfblk14 : Delay
  cfblk3 : Product
  cfblk4 : Reshape
  cfblk5 : Signum
  cfblk6 : Trigonometry
  cfblk7 : Assignment  DiagnosticForDimensions=Warning  IndexOptions=Index vector (dialog)  Indices=1  OutputSizes=1
  cfblk8 : Constant  Value=[23282084.198614]  SampleTime=1
  cfblk9 : Subsystem
  cfblk2 : Outport
  wires:
  cfblk7/1 -> cfblk3/1
  cfblk8/1 -> cfblk13/1(cfblk1), cfblk6/1
  cfblk4/1 -> cfblk7/2
  cfblk9/1(cfblk2) -> cfblk2/1
  cfblk12/1(cfblk2) -> cfblk10/1(cfblk1)
  cfblk6/1 -> cfblk9/1(cfblk1)
  cfblk11/1(cfblk2) -> cfblk3/2
  cfblk3/1 -> cfblk5/1
  cfblk10/1(cfblk2) -> cfblk11/1(cfblk1)
  cfblk13/1(cfblk2) -> cfblk12/1(cfblk1)
  cfblk1/1 -> cfblk4/1
  cfblk5/1 -> cfblk14/1
  cfblk14/1 -> cfblk7/1

== system sampleModel25/cfblk140/cfblk14 ==
  cfblk1 : Inport
  cfblk10 : Inport  Port=2
  cfblk11 : Inport  Port=3
  cfblk12 : Inport  Port=4
  Action Port : ActionPort  ActionType=else
  cfblk13 : Subsystem  TreatAsAtomicUnit=on
  cfblk14 : Subsystem  TreatAsAtomicUnit=on
  cfblk15 : Delay
  cfblk16 : Delay
  cfblk3 : Signum
  cfblk4 : Sin  TimeSource=Use external signal  SampleTime=0
  cfblk5 : Constant  Value=[492346463.790148]  SampleTime=1
  cfblk6 : Subsystem
  cfblk7 : Subsystem
  cfblk8 : Subsystem
  cfblk9 : If  IfExpression=u1 >= 0  SampleTime=1
  cfblk2 : Outport
  wires:
  cfblk13/1(cfblk2) -> cfblk7/1(cfblk1)
  cfblk1/1 -> cfblk4/1
  cfblk11/1 -> cfblk8/1(cfblk1)
  cfblk8/1(cfblk2) -> cfblk6/1(cfblk1)
  cfblk3/1 -> cfblk14/1(cfblk1)
  cfblk13/2(cfblk16) -> cfblk2/1
  cfblk5/1 -> cfblk9/1
  cfblk4/1 -> cfblk13/1(cfblk1)
  cfblk12/1 -> cfblk3/1
  cfblk9/1 -> cfblk13/Action
  cfblk9/2 -> cfblk14/Action
  cfblk7/1(cfblk2) -> cfblk15/1
  cfblk15/1 -> cfblk14/2(cfblk11)
  cfblk14/1(cfblk2) -> cfblk16/1
  cfblk16/1 -> cfblk13/2(cfblk15)

== system sampleModel25/cfblk140/cfblk15 ==
  cfblk1 : Inport
  Action Port : ActionPort  ActionType=then
  cfblk3 : DiscreteStateSpace  SampleTime=-1
  cfblk4 : PermuteDimensions
  cfblk5 : UnaryMinus
  cfblk6 : Sqrt  Operator=rSqrt  AlgorithmType=Newton-Raphson  SaturateOnIntegerOverflow=on
  cfblk7 : Constant  Value=[-555158907.269161]  SampleTime=1
  cfblk8 : Constant  Value=[-318230082.990717]  SampleTime=1
  cfblk9 : Subsystem
  cfblk2 : Outport
  wires:
  cfblk3/1 -> cfblk2/1
  cfblk6/1 -> cfblk9/1(cfblk1)
  cfblk5/1 -> cfblk4/1
  cfblk9/1(cfblk2) -> cfblk5/1
  cfblk7/1 -> cfblk6/1
  cfblk4/1 -> cfblk3/1

== system sampleModel25/cfblk140/cfblk16 ==
  cfblk1 : Inport
  Action Port : ActionPort  ActionType=else
  cfblk3 : DiscreteStateSpace  SampleTime=-1
  cfblk4 : DotProduct  InputSameDT=on  OutDataTypeStr=Inherit: Inherit via internal rule
  cfblk5 : Rounding
  cfblk6 : Subsystem
  cfblk7 : Subsystem
  cfblk2 : Outport
  cfblk8 : Outport  Port=2
  wires:
  cfblk3/1 -> cfblk4/1
  cfblk1/1 -> cfblk7/1(cfblk1)
  cfblk7/1(cfblk2) -> cfblk5/1
  cfblk5/1 -> cfblk3/1, cfblk4/2
  cfblk4/1 -> cfblk8/1, cfblk6/1(cfblk1)
  cfblk6/1(cfblk2) -> cfblk2/1

== system sampleModel25/cfblk140/cfblk7 ==
  cfblk1 : Inport
  cfblk2 : Outport
  wires:
  cfblk1/1 -> cfblk2/1

== system sampleModel25/cfblk140/cfblk8 ==
  cfblk1 : Inport
  cfblk2 : Outport
  wires:
  cfblk1/1 -> cfblk2/1

== system sampleModel25/cfblk140/cfblk9 ==
  cfblk1 : Inport
  cfblk2 : Outport
  wires:
  cfblk1/1 -> cfblk2/1

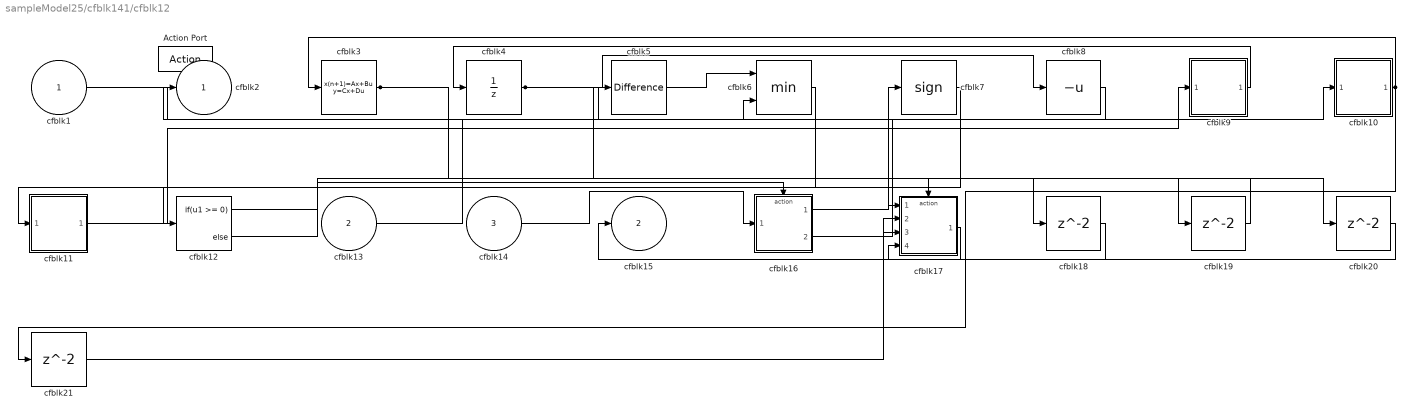
== system sampleModel25/cfblk141/cfblk12 ==
  cfblk1 : Inport
  cfblk13 : Inport  Port=2
  cfblk14 : Inport  Port=3
  Action Port : ActionPort  ActionType=then
  cfblk10 : Subsystem
  cfblk11 : Subsystem
  cfblk12 : If  IfExpression=u1 >= 0  SampleTime=1
  cfblk16 : Subsystem  TreatAsAtomicUnit=on
  cfblk17 : Subsystem  TreatAsAtomicUnit=on
  cfblk{18..21} (4 alike) : Delay
  cfblk3 : DiscreteStateSpace  SampleTime=-1
  cfblk4 : UnitDelay  SampleTime=-1
  cfblk5 : simulink/Discrete/Difference  ICPrevInput=0.0  OutMin=[]  OutMax=[]  OutDataTypeStr=Inherit: Inherit via back propagation  OutDataType=fixdt(1, 16)  OutScaling=2^-10  DoSatur=off
  cfblk6 : MinMax  Inputs=2
  cfblk7 : Signum
  cfblk8 : UnaryMinus
  cfblk9 : Subsystem
  cfblk2 : Outport
  cfblk15 : Outport  Port=2
  wires:
  cfblk4/1 -> cfblk8/1, cfblk18/1
  cfblk1/1 -> cfblk5/1
  cfblk17/1(cfblk2) -> cfblk15/1
  cfblk11/1(cfblk2) -> cfblk9/1(cfblk1)
  cfblk5/1 -> cfblk6/1
  cfblk9/1(cfblk2) -> cfblk4/1
  cfblk6/1 -> cfblk12/1
  cfblk10/1(cfblk2) -> cfblk3/1, cfblk21/1
  cfblk7/1 -> cfblk11/1(cfblk1)
  cfblk8/1 -> cfblk2/1
  cfblk13/1 -> cfblk6/2
  cfblk16/1(cfblk2) -> cfblk7/1
  cfblk14/1 -> cfblk16/1(cfblk1)
  cfblk16/2(cfblk9) -> cfblk10/1(cfblk1)
  cfblk3/1 -> cfblk19/1, cfblk20/1
  cfblk12/1 -> cfblk16/Action
  cfblk12/2 -> cfblk17/Action
  cfblk18/1 -> cfblk17/4(cfblk15)
  cfblk19/1 -> cfblk17/1(cfblk1)
  cfblk20/1 -> cfblk17/3(cfblk14)
  cfblk21/1 -> cfblk17/2(cfblk13)

== system sampleModel25/cfblk141/cfblk13 ==
  cfblk1 : Inport
  Action Port : ActionPort  ActionType=else
  cfblk10 : Subsystem
  cfblk11 : If  IfExpression=u1 >= 0  SampleTime=1
  cfblk12 : Subsystem  TreatAsAtomicUnit=on
  cfblk13 : Subsystem  TreatAsAtomicUnit=on
  cfblk{14..17} (4 alike) : Delay
  cfblk3 : DiscreteTransferFcn
  cfblk4 : DiscreteFir
  cfblk5 : Rounding
  cfblk6 : Constant  Value=[4742206.397453]  SampleTime=1
  cfblk7 : Subsystem
  cfblk8 : Subsystem
  cfblk9 : Subsystem
  cfblk2 : Outport
  wires:
  cfblk4/1 -> cfblk9/1(cfblk1), cfblk13/4(cfblk10)
  cfblk12/1(cfblk2) -> cfblk2/1
  cfblk8/1(cfblk2) -> cfblk3/1, cfblk12/2(cfblk16)
  cfblk10/1(cfblk2) -> cfblk11/1
  cfblk9/1(cfblk2) -> cfblk7/1(cfblk1)
  cfblk3/1 -> cfblk10/1(cfblk1)
  cfblk13/1(cfblk2) -> cfblk5/1
  cfblk6/1 -> cfblk8/1(cfblk1)
  cfblk5/1 -> cfblk14/1, cfblk15/1
  cfblk1/1 -> cfblk13/3(cfblk9)
  cfblk13/2(cfblk12) -> cfblk12/1(cfblk1)
  cfblk11/1 -> cfblk12/Action
  cfblk11/2 -> cfblk13/Action
  cfblk14/1 -> cfblk13/2(cfblk8)
  cfblk15/1 -> cfblk13/5(cfblk11)
  cfblk12/2(cfblk17) -> cfblk16/1
  cfblk16/1 -> cfblk13/1(cfblk1)
  cfblk7/1(cfblk2) -> cfblk17/1
  cfblk17/1 -> cfblk4/1
